simulink subsystem "Motores"  (R2023b)
settings: Solver=VariableStepAuto  StartTime=0.0  StopTime=10.0  RelTol=1e-3
libraries: arduinolib x6, simulink x2
settings Model: Creator=marqu  LastModifiedBy=marqu

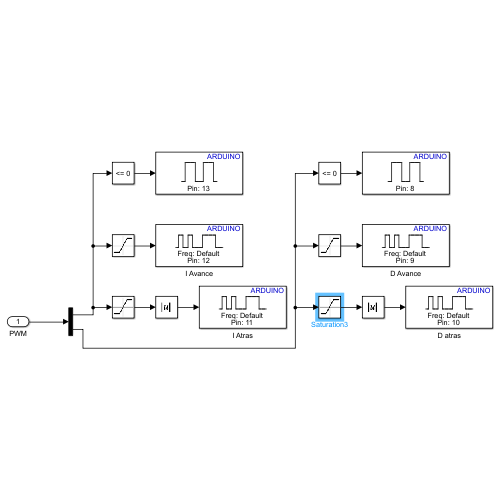
[thumbnail: Simulink's stored preview of the top-level diagram]
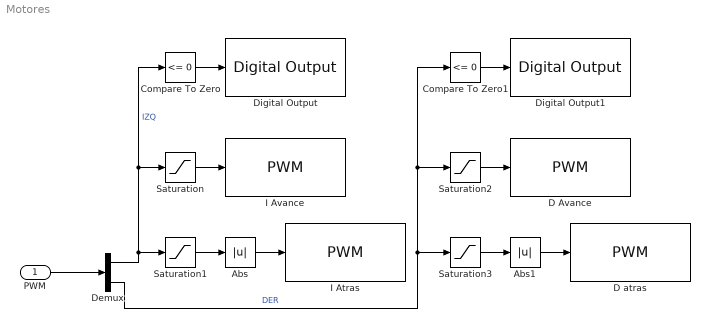
== system Motores ==
  PWM : Inport
  Abs : Abs  SaturateOnIntegerOverflow=off
  Abs1 : Abs  SaturateOnIntegerOverflow=off
  Compare To Zero : simulink/Logic and Bit Operations/Compare To Zero  relop=<=  OutDataTypeStr=boolean
  Compare To Zero1 : simulink/Logic and Bit Operations/Compare To Zero  relop=<=  OutDataTypeStr=boolean
  D Avance : arduinolib/PWM  pinNumber=9  frequencyType=Default  desiredFrequency=490.2  achievableFrequency=490.2
  D atras : arduinolib/PWM  pinNumber=10  frequencyType=Default  desiredFrequency=490.2  achievableFrequency=490.2
  Demux : Demux  Outputs=2
  Digital Output : arduinolib/Digital Output  pinNumber=13  Direction=output  blockPlatform=arduino
  Digital Output1 : arduinolib/Digital Output  pinNumber=8  Direction=output  blockPlatform=arduino
  I Atras : arduinolib/PWM  pinNumber=11  frequencyType=Default  desiredFrequency=490.2  achievableFrequency=490.2
  I Avance : arduinolib/PWM  pinNumber=12  frequencyType=Default  desiredFrequency=490.2  achievableFrequency=490.2
  Saturation : Saturate  UpperLimit=255  LowerLimit=0
  Saturation1 : Saturate  UpperLimit=0  LowerLimit=-255
  Saturation2 : Saturate  UpperLimit=255  LowerLimit=0
  Saturation3 : Saturate  UpperLimit=0  LowerLimit=-255
  wires:
  Demux/1 -> Saturation1/1, Saturation/1, Compare To Zero/1  "IZQ"
  Saturation/1 -> I Avance/1
  Compare To Zero/1 -> Digital Output/1
  Saturation1/1 -> Abs/1
  Abs/1 -> I Atras/1
  Demux/2 -> Saturation3/1, Saturation2/1, Compare To Zero1/1  "DER"
  Saturation2/1 -> D Avance/1
  Compare To Zero1/1 -> Digital Output1/1
  Saturation3/1 -> Abs1/1
  Abs1/1 -> D atras/1
  PWM/1 -> Demux/1
